simulink model "Sim_JointSpace"  (R2022b)
settings: Solver=ode1  StartTime=0.0  StopTime=Tf  FixedStep=t_step  RelTol=1e-3
undefined symbols (not defined in the file or in its folder): F, Im, Kd, Kp, kr, lx, ly, lz, mm, qt, rho, t_step
libraries: slpidlib x1
settings Model: Creator=vincenzo  LastModifiedBy=vincenzo

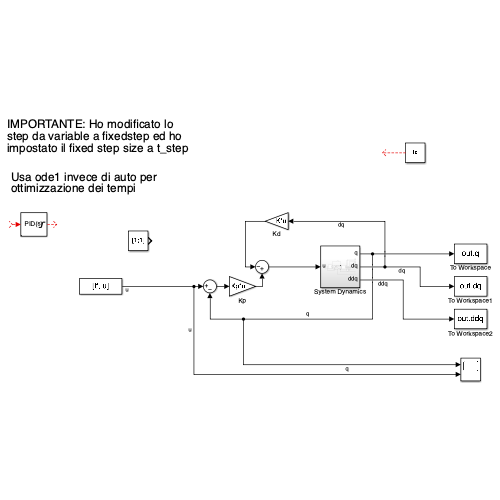
[thumbnail: Simulink's stored preview of the top-level diagram]
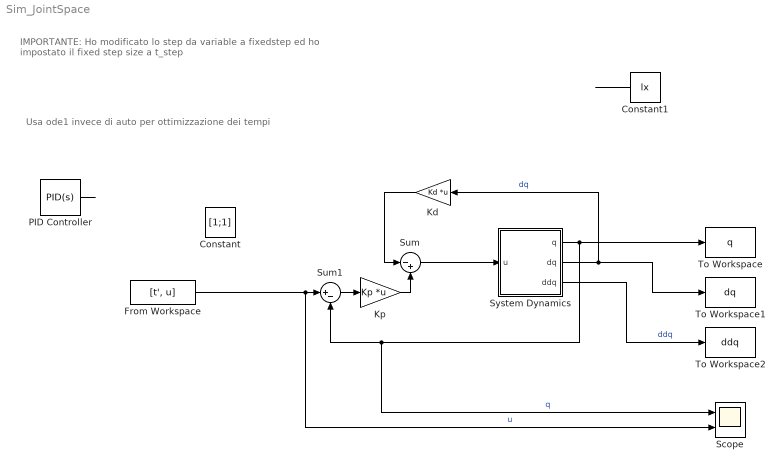
== system Sim_JointSpace ==
  note: Usa ode1 invece di auto per ottimizzazione dei tempi
  note: IMPORTANTE: Ho modificato lo step da variable a fixedstep ed ho impostato il fixed step size a t_step
  Constant : Constant  Value=[1;1]
  Constant1 : Constant  Value=lx
  From Workspace : FromWorkspace  VariableName=[t', u]  OutDataTypeStr=double  SampleTime=t_step
  Kd : Gain  Gain=Kd  Multiplication=Matrix(K*u)
  Kp : Gain  Gain=Kp  Multiplication=Matrix(K*u)
  PID Controller : slpidlib/PID Controller  Controller=PID  Form=Parallel  TimeDomain=Continuous-time  UseExternalTs=off  SampleTime=-1  IntegratorMethod=Forward Euler  FilterMethod=Forward Euler  ControllerParametersSource=internal  P=1/100  I=0  UseKiTs=off  D=0  N=100  UseFilter=on  TunerSelectOption=Transfer Function Based (PID Tuner App)  InitialConditionSource=internal  InitialConditionForIntegrator=0  InitialConditionForFilter=0  DifferentiatorICPrevScaledInput=0  ExternalReset=none  TrackingMode=off  Kt=1  LimitOutput=on  SatLimitsSource=internal  UpperSaturationLimit=4.5  LowerSaturationLimit=-4.5  LinearizeAsGain=on  AntiWindupMode=clamping  Kb=1  LimitIntegrator=off  UpperIntegratorSaturationLimit=inf  LowerIntegratorSaturationLimit=-inf  POutMin=[]  POutMax=[]  IOutMin=[]  IOutMax=[]  DOutMin=[]  DOutMax=[]  NOutMin=[]  NOutMax=[]  SumOutMin=[]  SumOutMax=[]  SaturationOutMin=[]  SaturationOutMax=[]  PParamMin=[]  PParamMax=[]  IParamMin=[]  IParamMax=[]  DParamMin=[]  DParamMax=[]  NParamMin=[]  NParamMax=[]  KbParamMin=[]  KbParamMax=[]  KtParamMin=[]  KtParamMax=[]  KbOutMin=[]  KbOutMax=[]  KtOutMin=[]  KtOutMax=[]  IntegratorOutMin=[]  IntegratorOutMax=[]  FilterOutMin=[]  FilterOutMax=[]  SumI1OutMin=[]  SumI1OutMax=[]  SumI2OutMin=[]  SumI2OutMax=[]  SumI3OutMin=[]  SumI3OutMax=[]  SumI4OutMin=[]  SumI4OutMax=[]  SumDOutMin=[]  SumDOutMax=[]  DifferentiatorOutMin=[]  DifferentiatorOutMax=[]  FilterDiffOutCoefMin=[]  FilterDiffOutCoefMax=[]  ReciprocalOutMin=[]  ReciprocalOutMax=[]  SumDenOutMin=[]  SumDenOutMax=[]  SumNumOutMin=[]  SumNumOutMax=[]  DivideOutMin=[]  DivideOutMax=[]  UdiffTsProdOutMin=[]  UdiffTsProdOutMax=[]  NTsProdOutMin=[]  NTsProdOutMax=[]  UintegralTsProdOutMin=[]  UintegralTsProdOutMax=[]  UngainTsProdOutMin=[]  UngainTsProdOutMax=[]  ClampingZeroOutDataTypeStr=Inherit: Inherit via back propagation  ClampingZeroOutMin=[]  ClampingZeroOutMax=[]  FilterDenConstantOutDataTypeStr=Inherit: Inherit via back propagation  FilterDenConstantOutMin=[]  FilterDenConstantOutMax=[]  PCopyOutDataTypeStr=Inherit: Inherit via back propagation  PCopyOutMin=[]  PCopyOutMax=[]  NCopyOutDataTypeStr=Inherit: Inherit via back propagation  NCopyOutMin=[]  NCopyOutMax=[]  IntegratorContinuousStateAttributes=''  IntegratorStateMustResolveToSignalObject=off  IntegratorRTWStateStorageClass=Auto  FilterContinuousStateAttributes=''  FilterStateMustResolveToSignalObject=off  FilterRTWStateStorageClass=Auto  ParallelPVariant=InternalParameters  IdealPVariant=Disabled  IVariant=InternalParameters  DVariant=InternalParameters  IntegratorVariant=Continuous  SatVariant=Enabled  AWVariant=ContClampingParallel  PCopyVariant=Disabled  TRVariant=Disabled  FdbkBlocksVariant=Forward  IdealPFdbkVariant=Disabled  SatFdbkVariant=Disabled  DerivativeFilterVariant=ContFilter  NVariant=InternalParameters  NCopyVariant=Disabled  FilterICVariant=InternalICsFilter  IntegratorICVariant=InternalICs  ExternalResetVariant=Disabled  TRSumVariant=Passthrough  SumFdbkVariant=Disabled  SumVariant=Sum_PID  TsampFilterVariant=InternalTs  TsampNgainVariant=Passthrough  TsampIntegralVariant=Passthrough  ExternalSaturationOutDataTypeStr=Inherit: Same as second input
  Scope : Scope  NumInputPorts=2
  Sum : Sum  Inputs=|-+
  Sum1 : Sum  Inputs=|+-
  System Dynamics : Subsystem
  To Workspace : ToWorkspace  VariableName=q  SampleTime=-1
      settings: Save2DSignal=2-D array (concatenate along first dimension)
  To Workspace1 : ToWorkspace  VariableName=dq  SampleTime=-1
      settings: Save2DSignal=2-D array (concatenate along first dimension)
  To Workspace2 : ToWorkspace  VariableName=ddq  SampleTime=-1
      settings: Save2DSignal=2-D array (concatenate along first dimension)
  wires:
  ? -> PID Controller/1
  System Dynamics/1(q) -> Scope/1, Sum1/2, To Workspace/1  "q"
  PID Controller/1 -> ?
  System Dynamics/2(dq) -> Kd/1, To Workspace1/1  "dq"
  System Dynamics/3(ddq) -> To Workspace2/1  "ddq"
  Sum1/1 -> Kp/1
  Kp/1 -> Sum/2
  Kd/1 -> Sum/1
  Sum/1 -> System Dynamics/1(u)
  Constant1/1 -> ?
  From Workspace/1 -> Scope/2, Sum1/1  "u"

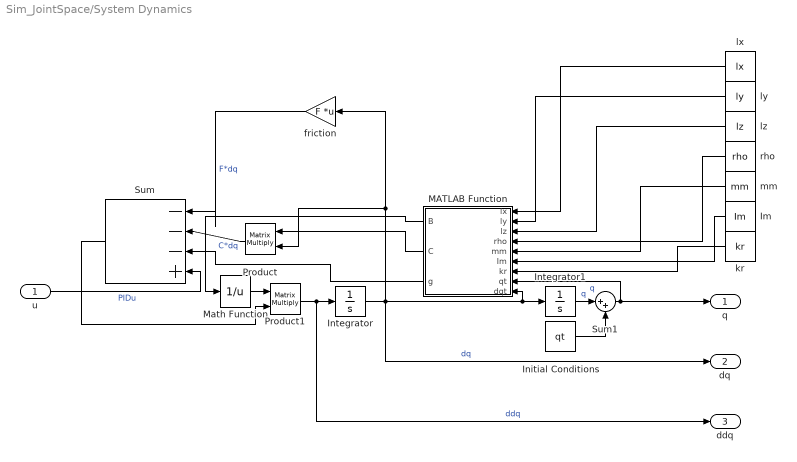
== system Sim_JointSpace/System Dynamics ==
  u : Inport
  Im : Constant  Value=Im
  Initial Conditions : Constant  Value=qt
  Integrator : Integrator  InitialCondition=[0; 0]
  Integrator1 : Integrator  InitialCondition=[0;0]
  MATLAB Function : MATLAB Function  TreatAsAtomicUnit=on
  Math Function : Math  Operator=reciprocal
  Product : Product  Multiplication=Matrix(*)
  Product1 : Product  Multiplication=Matrix(*)
  Sum : Sum  Inputs=|---+
  Sum1 : Sum  Inputs=|++
  friction : Gain  Gain=F  Multiplication=Matrix(K*u)
  kr : Constant  Value=kr
  lx : Constant  Value=lx
  ly : Constant  Value=ly
  lz : Constant  Value=lz
  mm : Constant  Value=mm
  rho : Constant  Value=rho
  q : Outport
  dq : Outport  Port=2
  ddq : Outport  Port=3
  wires:
  Sum/1 -> Product1/2
  friction/1 -> Sum/1  "F*dq"
  MATLAB Function/1(B) -> Math Function/1
  Sum1/1 -> MATLAB Function/8(qt), q/1  "q"
  lx/1 -> MATLAB Function/1(lx)
  MATLAB Function/2(C) -> Product/1
  Product/1 -> Sum/2  "C*dq"
  Math Function/1 -> Product1/1
  ly/1 -> MATLAB Function/2(ly)
  Integrator/1 -> dq/1, Integrator1/1, MATLAB Function/9(dqt), Product/2, friction/1  "dq"
  Product1/1 -> ddq/1, Integrator/1  "ddq"
  MATLAB Function/3(g) -> Sum/3
  lz/1 -> MATLAB Function/3(lz)
  mm/1 -> MATLAB Function/5(mm)
  kr/1 -> MATLAB Function/7(kr)
  rho/1 -> MATLAB Function/4(rho)
  Im/1 -> MATLAB Function/6(Im)
  u/1 -> Sum/4  "PIDu"
  Integrator1/1 -> Sum1/1  "q"
  Initial Conditions/1 -> Sum1/2

== matlab function Sim_JointSpace/System Dynamics/MATLAB Function ==
  data: lx input; ly input; lz input; rho input; mm input; Im input; kr input; qt input; B output; dqt input; C output; g output
function [B, C, g] = fcn(lx, ly, lz, rho, mm, Im, kr, qt, dqt)
coder.extrinsic('generateBCg');
B = zeros(2);
C = zeros(2);
g = zeros(2,1);
[B, C, g] = generateBCg(lx, ly, lz, rho, mm, Im, kr, qt, dqt);
